simulink model "inverse"  (R2019a)
settings: Solver=VariableStepAuto  StartTime=0.0  StopTime=10.0  RelTol=1e-3
settings Model: Creator=COMPUMARTS  LastModifiedBy=COMPUMARTS

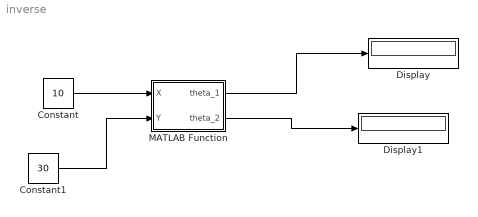
== system inverse ==
  Constant : Constant  Value=10
  Constant1 : Constant  Value=30
  Display : Display
  Display1 : Display
  MATLAB Function : MATLAB Function  TreatAsAtomicUnit=on
  wires:
  Constant/1 -> MATLAB Function/1(X)
  Constant1/1 -> MATLAB Function/2(Y)
  MATLAB Function/1(theta_1) -> Display/1
  MATLAB Function/2(theta_2) -> Display1/1

== matlab function inverse/MATLAB Function ==
  data: X input; theta_1 output; Y input; theta_2 output

function [theta_1,theta_2] = fcn(X, Y)

    lenth = 0.25;
    lenth_6 = 0.2;
    theta_1=0;
    theta_2=0;
    val=50;
    val_2=50;
    
    
    X=X/100;
    Y=Y/100;
    K1 = sqrt(((X+(lenth_6/2))^2)+(Y^2));
    K2 = sqrt(((X-(lenth_6/2))^2)+(Y^2));
    
    if K1 ~= 0
        if K2 ~=0 
            val= ((K1^2)/(2*lenth*K1));
            val_2= ((K2^2)/(2*lenth*K2));
        end
    end
    if(val < 1)
        if (val > -1)
            if (val_2<1)
                if (val_2>-1)
                    pthai_1 = acos((K1^2)/(2*lenth*K1));
                    pthai_2 = acos((K2^2)/(2*lenth*K2));
    
                    zeta_1 = atan2(Y,(X+(lenth_6/2)));
                    zeta_2 = atan2(Y,(X-(lenth_6/2)));
    
                    theta_1 = rad2deg(zeta_1 + pthai_1);  
                    theta_2 = rad2deg(zeta_2 - pthai_2);
                   
                end
            end
        end
    end
